simulink model "c29_1"  (R2024a)
settings: Solver=VariableStepAuto  StartTime=0.0  StopTime=10.0  RelTol=1e-3
settings Model: Creator=17760  LastModifiedBy=17760

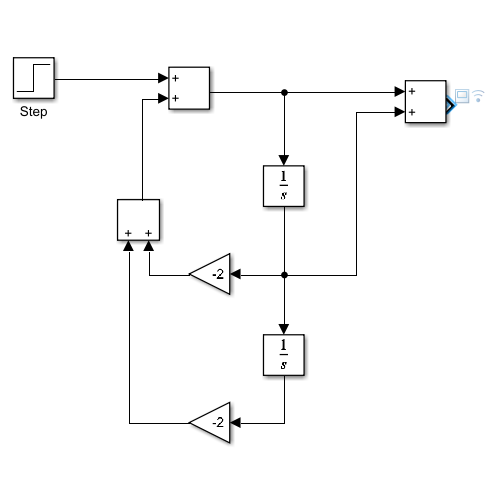
[thumbnail: Simulink's stored preview of the top-level diagram]
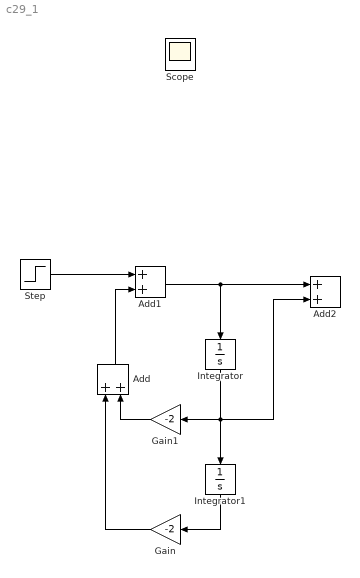
== system c29_1 ==
  Add : Sum
  Add1 : Sum
  Add2 : Sum
  Gain : Gain  Gain=-2
  Gain1 : Gain  Gain=-2
  Integrator : Integrator
  Integrator1 : Integrator
  Step : Step  SampleTime=0
  Scope : Scope
  wires:
  Integrator/1 -> Gain1/1, Integrator1/1, Add2/2
  Integrator1/1 -> Gain/1
  Gain/1 -> Add/1
  Step/1 -> Add1/1
  Add/1 -> Add1/2
  Gain1/1 -> Add/2
  Add1/1 -> Integrator/1, Add2/1
